simulink model "motor"  (Simulink 8.6)
settings: Solver=FixedStepDiscrete  StartTime=0.0  StopTime=inf  FixedStep=0.002  RelTol=1e-3
PostLoadFcn:
  | ,try, rti_mdl_postloadfcn(bdroot, 'UpdateModel', 160, 'rti1104'); catch, disp(lasterr); end,
undefined symbols (not defined in the file): DiscIntNeverNeededParam
libraries: simulink x3
(part 2 of 3)

== system motor/Chart/Motor_XHHY/Control_HP ==
  In_HP : Inport
  Discrete-Time Integrator : DiscreteIntegrator  InitialConditionSetting=State (most efficient)  SampleTime=-1  ICPrevOutput=DiscIntNeverNeededParam  ICPrevScaledInput=DiscIntNeverNeededParam
  KD_KG : Gain  Gain=0
  P_KP : DataStoreRead  DataStoreName=P_KP
  Product : Product
  Sum : Sum  Inputs=|+-
  Sum1 : Sum  Inputs=|++
  ZP_KN : Gain  Gain=100
  ZP_Kp1 : Gain
  ZP_Kp2 : Gain  Gain=0.001
  ZV_KD1 : Gain  Gain=0.036
  Out_HP : Outport
  wires:
  Product/1 -> ZP_Kp1/1, ZP_Kp2/1
  ZP_Kp2/1 -> ZV_KD1/1
  ZV_KD1/1 -> Sum/1
  Sum/1 -> ZP_KN/1
  Discrete-Time Integrator/1 -> Sum/2
  ZP_Kp1/1 -> Sum1/1
  Sum1/1 -> Out_HP/1
  KD_KG/1 -> Sum1/2
  ZP_KN/1 -> Discrete-Time Integrator/1, KD_KG/1
  In_HP/1 -> Product/1
  P_KP/1 -> Product/2

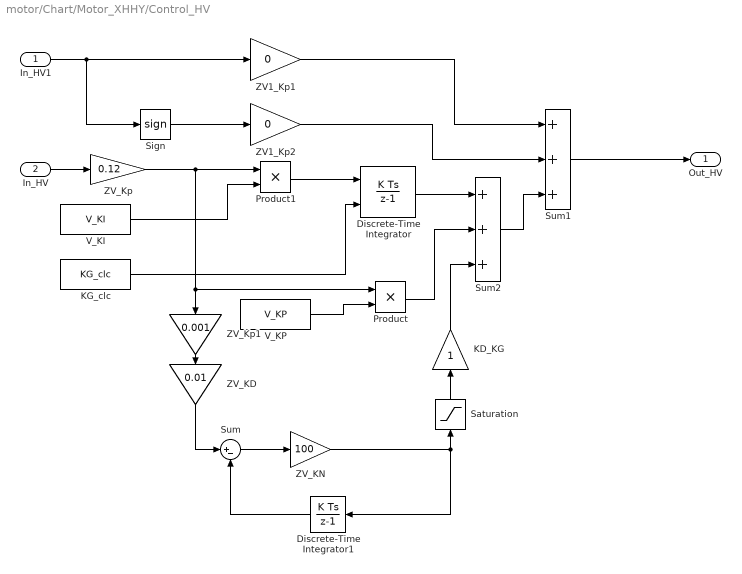
== system motor/Chart/Motor_XHHY/Control_HV ==
  In_HV1 : Inport
  In_HV : Inport  Port=2
  Discrete-Time Integrator : DiscreteIntegrator  ExternalReset=either  SampleTime=-1  SaturateOnIntegerOverflow=on  LimitOutput=on  UpperSaturationLimit=2000  LowerSaturationLimit=-2000  ICPrevOutput=DiscIntNeverNeededParam  ICPrevScaledInput=DiscIntNeverNeededParam
  Discrete-Time Integrator1 : DiscreteIntegrator  InitialConditionSetting=State (most efficient)  SampleTime=-1  LimitOutput=on  UpperSaturationLimit=2000  LowerSaturationLimit=-2000  ICPrevOutput=DiscIntNeverNeededParam  ICPrevScaledInput=DiscIntNeverNeededParam
  KD_KG : Gain
  KG_clc : DataStoreRead  DataStoreName=KG_clc
  Product : Product
  Product1 : Product
  Saturation : Saturate  UpperLimit=300  LowerLimit=-300
  Sign : Signum
  Sum : Sum  Inputs=|+-
  Sum1 : Sum  Inputs=+++
  Sum2 : Sum  Inputs=+++
  V_KI : DataStoreRead  DataStoreName=V_KI
  V_KP : DataStoreRead  DataStoreName=V_KP
  ZV1_Kp1 : Gain  Gain=0
  ZV1_Kp2 : Gain  Gain=0
  ZV_KD : Gain  Gain=0.01
  ZV_KN : Gain  Gain=100
  ZV_Kp : Gain  Gain=0.12
  ZV_Kp1 : Gain  Gain=0.001
  Out_HV : Outport
  wires:
  Product/1 -> Sum2/2
  Discrete-Time Integrator/1 -> Sum2/1
  In_HV/1 -> ZV_Kp/1
  Sign/1 -> ZV1_Kp2/1
  In_HV1/1 -> Sign/1, ZV1_Kp1/1
  Sum1/1 -> Out_HV/1
  Sum2/1 -> Sum1/3
  ZV1_Kp2/1 -> Sum1/2
  ZV1_Kp1/1 -> Sum1/1
  ZV_Kp1/1 -> ZV_KD/1
  ZV_KD/1 -> Sum/1
  Sum/1 -> ZV_KN/1
  Discrete-Time Integrator1/1 -> Sum/2
  ZV_KN/1 -> Discrete-Time Integrator1/1, Saturation/1
  Saturation/1 -> KD_KG/1
  KD_KG/1 -> Sum2/3
  KG_clc/1 -> Discrete-Time Integrator/2
  Product1/1 -> Discrete-Time Integrator/1
  ZV_Kp/1 -> ZV_Kp1/1, Product/1, Product1/1
  V_KP/1 -> Product/2
  V_KI/1 -> Product1/2

== system motor/Chart/Motor_XHHY/If Action Subsystem1 ==
  Action Port : ActionPort  ActionType=elseif
  Data Store Read : DataStoreRead  DataStoreName=JD_XHHY_HC
  Data Store Write1 : DataStoreWrite  DataStoreName=JD_XHHY
  wires:
  Data Store Read/1 -> Data Store Write1/1

== system motor/Chart/Motor_XHHY/If Action Subsystem2 ==
  In1 : Inport
  Action Port : ActionPort  ActionType=else
  Data Store Write : DataStoreWrite  DataStoreName=JD_XHHY_HC
  Data Store Write1 : DataStoreWrite  DataStoreName=JD_XHHY
  wires:
  In1/1 -> Data Store Write/1, Data Store Write1/1

== system motor/Chart/Motor_XHHY/If Action Subsystem3 ==
  In1 : Inport
  Action Port : ActionPort  ActionType=then
  Data Store Write : DataStoreWrite  DataStoreName=JD_XHHY_HC
  Data Store Write1 : DataStoreWrite  DataStoreName=JD_XHHY
  wires:
  In1/1 -> Data Store Write/1, Data Store Write1/1

== system motor/Chart/Motor_XHHY/Switch Case Action Subsystem ==
  In1 : Inport
  Action Port : ActionPort  ActionType=then
  Constant : Constant  Value=0
  Data Store Write : DataStoreWrite  DataStoreName=Angle_extern
  Data Store Write1 : DataStoreWrite  DataStoreName=Angle_internal
  wires:
  In1/1 -> Data Store Write/1
  Constant/1 -> Data Store Write1/1

== system motor/Chart/Motor_XHHY/Switch Case Action Subsystem1 ==
  In1 : Inport
  Action Port : ActionPort  ActionType=else
  Constant : Constant  Value=0
  Data Store Write : DataStoreWrite  DataStoreName=Angle_extern
  Data Store Write1 : DataStoreWrite  DataStoreName=Angle_internal
  wires:
  In1/1 -> Data Store Write1/1
  Constant/1 -> Data Store Write/1

== system motor/Chart/Motor_XHHY/ZYDX_XHHY ==
  Hl : Inport  OutDataTypeStr=double
  Zl : Inport  Port=2  OutDataTypeStr=double
  Fcn1 : Fcn  Expr=u+265.5
  Fcn10 : Fcn  Expr=u*u+1
  Fcn11 : Fcn  Expr=sqrt(u)
  Fcn12 : Fcn  Expr=2*atan(u)
  Fcn2 : Fcn  Expr=(90490.25-u*u)/(20000)
  Fcn3 : Fcn  Expr=(2.655-sqrt(2.655*2.655-u*u+1))/(u+1)
  Fcn4 : Fcn  Expr=2.655*cos(u)
  Fcn5 : Fcn  Expr=u+265.5
  Fcn6 : Fcn  Expr=2*atan(u)
  Fcn7 : Fcn  Expr=(90490.25-u*u)/(20000)
  Fcn8 : Fcn  Expr=u*u
  Fcn9 : Fcn  Expr=1/(u+1)
  Product : Product  RndMeth=Zero
  Sum2 : Sum  Inputs=|+-
  Sum3 : Sum  Inputs=|+-
  Hq : Outport
  wires:
  Fcn11/1 -> Sum2/2
  Fcn4/1 -> Fcn10/1, Sum2/1
  Fcn3/1 -> Fcn6/1
  Hl/1 -> Fcn5/1
  Fcn1/1 -> Fcn2/1
  Product/1 -> Fcn12/1
  Fcn12/1 -> Hq/1
  Fcn2/1 -> Fcn3/1
  Fcn7/1 -> Fcn9/1, Fcn8/1
  Fcn6/1 -> Fcn4/1
  Zl/1 -> Fcn1/1
  Sum2/1 -> Product/1
  Fcn10/1 -> Sum3/1
  Fcn5/1 -> Fcn7/1
  Sum3/1 -> Fcn11/1
  Fcn9/1 -> Product/2
  Fcn8/1 -> Sum3/2

== system motor/Chart/Motor_XHZY/Control_ZP ==
  In_ZP : Inport
  Discrete-Time Integrator : DiscreteIntegrator  InitialConditionSetting=State (most efficient)  SampleTime=-1  ICPrevOutput=DiscIntNeverNeededParam  ICPrevScaledInput=DiscIntNeverNeededParam
  KD_KG : Gain  Gain=0
  P_KP : DataStoreRead  DataStoreName=P_KP
  Product : Product
  Sum : Sum  Inputs=|+-
  Sum1 : Sum  Inputs=|++
  ZP_KN : Gain  Gain=100
  ZP_Kp1 : Gain
  ZP_Kp2 : Gain  Gain=0.001
  ZV_KD1 : Gain  Gain=0.036
  Out_ZP : Outport
  wires:
  Product/1 -> ZP_Kp1/1, ZP_Kp2/1
  ZP_Kp2/1 -> ZV_KD1/1
  ZV_KD1/1 -> Sum/1
  Sum/1 -> ZP_KN/1
  Discrete-Time Integrator/1 -> Sum/2
  ZP_Kp1/1 -> Sum1/1
  Sum1/1 -> Out_ZP/1
  KD_KG/1 -> Sum1/2
  ZP_KN/1 -> Discrete-Time Integrator/1, KD_KG/1
  In_ZP/1 -> Product/1
  P_KP/1 -> Product/2

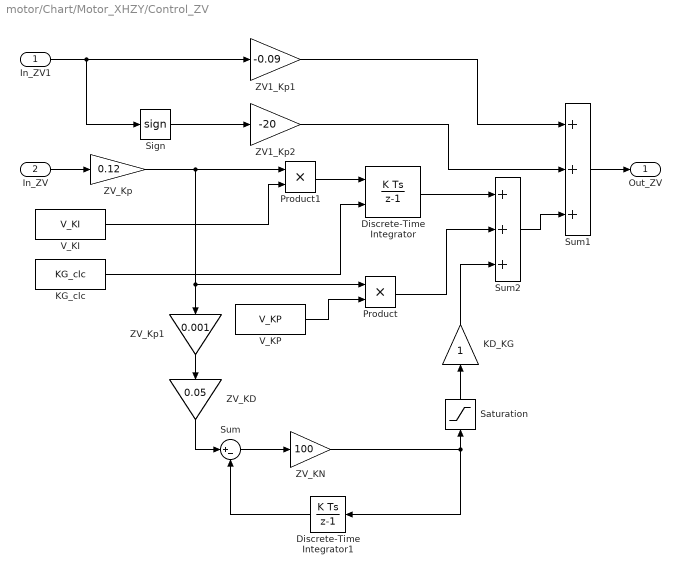
== system motor/Chart/Motor_XHZY/Control_ZV ==
  In_ZV1 : Inport
  In_ZV : Inport  Port=2
  Discrete-Time Integrator : DiscreteIntegrator  ExternalReset=either  SampleTime=-1  SaturateOnIntegerOverflow=on  LimitOutput=on  UpperSaturationLimit=2000  LowerSaturationLimit=-2000  ICPrevOutput=DiscIntNeverNeededParam  ICPrevScaledInput=DiscIntNeverNeededParam
  Discrete-Time Integrator1 : DiscreteIntegrator  InitialConditionSetting=State (most efficient)  SampleTime=-1  ICPrevOutput=DiscIntNeverNeededParam  ICPrevScaledInput=DiscIntNeverNeededParam
  KD_KG : Gain
  KG_clc : DataStoreRead  DataStoreName=KG_clc
  Product : Product
  Product1 : Product
  Saturation : Saturate  UpperLimit=300  LowerLimit=-300
  Sign : Signum
  Sum : Sum  Inputs=|+-
  Sum1 : Sum  Inputs=+++
  Sum2 : Sum  Inputs=+++
  V_KI : DataStoreRead  DataStoreName=V_KI
  V_KP : DataStoreRead  DataStoreName=V_KP
  ZV1_Kp1 : Gain  Gain=-0.09
  ZV1_Kp2 : Gain  Gain=-20
  ZV_KD : Gain  Gain=0.05
  ZV_KN : Gain  Gain=100
  ZV_Kp : Gain  Gain=0.12
  ZV_Kp1 : Gain  Gain=0.001
  Out_ZV : Outport
  wires:
  Product/1 -> Sum2/2
  Discrete-Time Integrator/1 -> Sum2/1
  In_ZV/1 -> ZV_Kp/1
  Sign/1 -> ZV1_Kp2/1
  In_ZV1/1 -> Sign/1, ZV1_Kp1/1
  Sum1/1 -> Out_ZV/1
  Sum2/1 -> Sum1/3
  ZV1_Kp2/1 -> Sum1/2
  ZV1_Kp1/1 -> Sum1/1
  ZV_Kp1/1 -> ZV_KD/1
  ZV_KD/1 -> Sum/1
  Sum/1 -> ZV_KN/1
  Discrete-Time Integrator1/1 -> Sum/2
  ZV_KN/1 -> Discrete-Time Integrator1/1, Saturation/1
  Saturation/1 -> KD_KG/1
  KD_KG/1 -> Sum2/3
  KG_clc/1 -> Discrete-Time Integrator/2
  Product1/1 -> Discrete-Time Integrator/1
  ZV_Kp/1 -> ZV_Kp1/1, Product/1, Product1/1
  V_KP/1 -> Product/2
  V_KI/1 -> Product1/2

== system motor/Chart/Motor_XHZY/If Action Subsystem1 ==
  Action Port : ActionPort  ActionType=elseif
  Data Store Read : DataStoreRead  DataStoreName=JD_XHZY_HC
  Data Store Read1 : DataStoreRead  DataStoreName=YJ_XHZY_HC
  Data Store Write1 : DataStoreWrite  DataStoreName=JD_XHZY
  Data Store Write2 : DataStoreWrite  DataStoreName=YJ_XHZY
  wires:
  Data Store Read/1 -> Data Store Write1/1
  Data Store Read1/1 -> Data Store Write2/1

== system motor/Chart/Motor_XHZY/If Action Subsystem2 ==
  In1 : Inport
  In2 : Inport  Port=2
  Action Port : ActionPort  ActionType=else
  Data Store Write : DataStoreWrite  DataStoreName=JD_XHZY_HC
  Data Store Write1 : DataStoreWrite  DataStoreName=JD_XHZY
  Data Store Write2 : DataStoreWrite  DataStoreName=YJ_XHZY_HC
  Data Store Write3 : DataStoreWrite  DataStoreName=YJ_XHZY
  wires:
  In1/1 -> Data Store Write/1, Data Store Write1/1
  In2/1 -> Data Store Write3/1, Data Store Write2/1

== system motor/Chart/Motor_XHZY/If Action Subsystem3 ==
  In1 : Inport
  In2 : Inport  Port=2
  Action Port : ActionPort  ActionType=then
  Data Store Write : DataStoreWrite  DataStoreName=JD_XHZY_HC
  Data Store Write1 : DataStoreWrite  DataStoreName=JD_XHZY
  Data Store Write2 : DataStoreWrite  DataStoreName=YJ_XHZY_HC
  Data Store Write3 : DataStoreWrite  DataStoreName=YJ_XHZY
  wires:
  In1/1 -> Data Store Write/1, Data Store Write1/1
  In2/1 -> Data Store Write3/1, Data Store Write2/1

== system motor/Chart/Motor_XHZY/Switch Case Action Subsystem ==
  In1 : Inport
  Action Port : ActionPort  ActionType=then
  Constant : Constant  Value=0
  Data Store Write : DataStoreWrite  DataStoreName=Angle_extern
  Data Store Write1 : DataStoreWrite  DataStoreName=Angle_internal
  wires:
  In1/1 -> Data Store Write/1
  Constant/1 -> Data Store Write1/1

== system motor/Chart/Motor_XHZY/Switch Case Action Subsystem1 ==
  In1 : Inport
  Action Port : ActionPort  ActionType=else
  Constant : Constant  Value=0
  Data Store Write : DataStoreWrite  DataStoreName=Angle_extern
  Data Store Write1 : DataStoreWrite  DataStoreName=Angle_internal
  wires:
  In1/1 -> Data Store Write1/1
  Constant/1 -> Data Store Write/1

== system motor/Chart/Motor_XHZY/ZYDX_XHZY ==
  Zl : Inport
  Fcn1 : Fcn  Expr=u+265.5
  Fcn2 : Fcn  Expr=(90490.25-u*u)/(20000)
  Fcn3 : Fcn  Expr=(2.655-sqrt(2.655*2.655-u*u+1))/(u+1)
  Fcn6 : Fcn  Expr=2*atan(u)
  Zq : Outport
  wires:
  Fcn3/1 -> Fcn6/1
  Zl/1 -> Fcn1/1
  Fcn6/1 -> Zq/1
  Fcn1/1 -> Fcn2/1
  Fcn2/1 -> Fcn3/1

== system motor/Chart/Open_Motor/sudu_PI ==
  In_ZV : Inport
  Discrete-Time Integrator : DiscreteIntegrator  ExternalReset=either  SampleTime=-1  SaturateOnIntegerOverflow=on  LimitOutput=on  UpperSaturationLimit=1000  LowerSaturationLimit=-1000  ICPrevOutput=DiscIntNeverNeededParam  ICPrevScaledInput=DiscIntNeverNeededParam
  Discrete-Time Integrator1 : DiscreteIntegrator  InitialConditionSetting=State (most efficient)  SampleTime=-1  ICPrevOutput=DiscIntNeverNeededParam  ICPrevScaledInput=DiscIntNeverNeededParam
  KD_KG : Gain  Gain=0
  KG_clc : DataStoreRead  DataStoreName=KG_clc
  Saturation : Saturate  UpperLimit=300  LowerLimit=-300
  Sum : Sum  Inputs=|+-
  Sum2 : Sum  Inputs=|+++
  ZV_KD : Gain  Gain=0.095
  ZV_KN : Gain  Gain=100
  ZV_Ki : Gain  Gain=0
  ZV_Kp : Gain  Gain=0.7
  ZV_Kp1 : Gain  Gain=0.001
  ZV_Kpt : Gain
  Out_ZV : Outport
  wires:
  ZV_Kpt/1 -> Sum2/2
  Discrete-Time Integrator/1 -> Sum2/1
  In_ZV/1 -> ZV_Kp/1
  ZV_Kp/1 -> ZV_Ki/1, ZV_Kp1/1, ZV_Kpt/1
  Sum2/1 -> Out_ZV/1
  ZV_Kp1/1 -> ZV_KD/1
  ZV_KD/1 -> Sum/1
  Sum/1 -> ZV_KN/1
  Discrete-Time Integrator1/1 -> Sum/2
  ZV_KN/1 -> Saturation/1, Discrete-Time Integrator1/1
  Saturation/1 -> KD_KG/1
  KD_KG/1 -> Sum2/3
  KG_clc/1 -> Discrete-Time Integrator/2
  ZV_Ki/1 -> Discrete-Time Integrator/1

== system motor/Chart/Waveform_Build/If Action Subsystem1 ==
  In1 : Inport
  In2 : Inport  Port=2
  Action Port : ActionPort  ActionType=then
  Data Store Read5 : DataStoreRead  DataStoreName=T_Count
  Data Store Write1 : DataStoreWrite  DataStoreName=T_Count
  Data Store Write2 : DataStoreWrite  DataStoreName=Temp1
  Data Store Write3 : DataStoreWrite  DataStoreName=T
  MATLAB Function : MATLAB Function  TreatAsAtomicUnit=on
  Out1 : Outport
  wires:
  In1/1 -> Out1/1
  In2/1 -> Data Store Write2/1
  MATLAB Function/1(y1) -> Data Store Write3/1
  Data Store Read5/1 -> MATLAB Function/1(u)
  MATLAB Function/2(y2) -> Data Store Write1/1

== system motor/Chart/Waveform_Build/If Action Subsystem2 ==
  In1 : Inport
  In2 : Inport  Port=2
  Action Port : ActionPort  ActionType=then
  Data Store Write2 : DataStoreWrite  DataStoreName=Temp2
  Out1 : Outport
  wires:
  In2/1 -> Data Store Write2/1
  In1/1 -> Out1/1

== system motor/Chart/Waveform_Build/If Action Subsystem3 ==
  Action Port : ActionPort  ActionType=else
  Add20 : Sum
  Constant3 : Constant
  Data Store Read5 : DataStoreRead  DataStoreName=T_Count
  Data Store Write1 : DataStoreWrite  DataStoreName=T_Count
  Saturation : Saturate  UpperLimit=999  LowerLimit=0
  Scope4 : Scope
  wires:
  Add20/1 -> Saturation/1
  Data Store Read5/1 -> Add20/1
  Constant3/1 -> Add20/2
  Saturation/1 -> Scope4/1, Data Store Write1/1

== system motor/Chart/Waveform_Build/If Action Subsystem4 ==
  In1 : Inport
  Action Port : ActionPort  ActionType=then
  Out1 : Outport
  wires:
  In1/1 -> Out1/1

== system motor/Chart/Angle_Calculation/If Action Subsystem1/ZYDX_HYDG ==
  l2 : Inport
  Cl1 : Fcn  Expr=(2*0.1*0.1+0.2655*0.2655-u*u)/(2*0.1*0.1)
  Fcn : Fcn  Expr=(2.655-sqrt(2.655*2.655-u*u+1))/(u+1)
  Fcn4 : Fcn  Expr=2*atan(u)
  Fcn7 : Fcn  Expr=u+0.2655
  x : Outport
  wires:
  Fcn4/1 -> x/1
  l2/1 -> Fcn7/1
  Fcn/1 -> Fcn4/1
  Fcn7/1 -> Cl1/1
  Cl1/1 -> Fcn/1

== system motor/Chart/Angle_Calculation/If Action Subsystem2/ZYDX_XHZY ==
  Zl : Inport
  Fcn1 : Fcn  Expr=u+265.5
  Fcn2 : Fcn  Expr=(90490.25-u*u)/(20000)
  Fcn3 : Fcn  Expr=(2.655-sqrt(2.655*2.655-u*u+1))/(u+1)
  Fcn6 : Fcn  Expr=2*atan(u)
  Zq : Outport
  wires:
  Fcn3/1 -> Fcn6/1
  Zl/1 -> Fcn1/1
  Fcn6/1 -> Zq/1
  Fcn1/1 -> Fcn2/1
  Fcn2/1 -> Fcn3/1

== system motor/Chart/Angle_Calculation/If Action Subsystem3/ZYDX_XHHY ==
  Hl : Inport  OutDataTypeStr=double
  Zl : Inport  Port=2  OutDataTypeStr=double
  Fcn1 : Fcn  Expr=u+265.5
  Fcn10 : Fcn  Expr=u*u+1
  Fcn11 : Fcn  Expr=sqrt(u)
  Fcn12 : Fcn  Expr=2*atan(u)
  Fcn2 : Fcn  Expr=(90490.25-u*u)/(20000)
  Fcn3 : Fcn  Expr=(2.655-sqrt(2.655*2.655-u*u+1))/(u+1)
  Fcn4 : Fcn  Expr=2.655*cos(u)
  Fcn5 : Fcn  Expr=u+265.5
  Fcn6 : Fcn  Expr=2*atan(u)
  Fcn7 : Fcn  Expr=(90490.25-u*u)/(20000)
  Fcn8 : Fcn  Expr=u*u
  Fcn9 : Fcn  Expr=1/(u+1)
  Product : Product  RndMeth=Zero
  Sum2 : Sum  Inputs=|+-
  Sum3 : Sum  Inputs=|+-
  Hq : Outport
  wires:
  Fcn11/1 -> Sum2/2
  Fcn4/1 -> Fcn10/1, Sum2/1
  Fcn3/1 -> Fcn6/1
  Hl/1 -> Fcn5/1
  Fcn1/1 -> Fcn2/1
  Product/1 -> Fcn12/1
  Fcn12/1 -> Hq/1
  Fcn2/1 -> Fcn3/1
  Fcn7/1 -> Fcn9/1, Fcn8/1
  Fcn6/1 -> Fcn4/1
  Zl/1 -> Fcn1/1
  Sum2/1 -> Product/1
  Fcn10/1 -> Sum3/1
  Fcn5/1 -> Fcn7/1
  Sum3/1 -> Fcn11/1
  Fcn9/1 -> Product/2
  Fcn8/1 -> Sum3/2

== system motor/Chart/Angle_Calculation_HY/fs_plat/ZYDX_HYDG ==
  l2 : Inport
  Cl1 : Fcn  Expr=(2*0.1*0.1+0.2655*0.2655-u*u)/(2*0.1*0.1)
  Fcn : Fcn  Expr=(2.655-sqrt(2.655*2.655-u*u+1))/(u+1)
  Fcn4 : Fcn  Expr=2*atan(u)
  Fcn7 : Fcn  Expr=u+0.2655
  x : Outport
  wires:
  Fcn4/1 -> x/1
  l2/1 -> Fcn7/1
  Fcn/1 -> Fcn4/1
  Fcn7/1 -> Cl1/1
  Cl1/1 -> Fcn/1

== system motor/Chart/BJ/If Action Subsystem/If Action Subsystem ==
  Action Port : ActionPort  ActionType=then
  Data Store Write : DataStoreWrite  DataStoreName=PC1
  Data Store Write1 : DataStoreWrite  DataStoreName=PC2
  Data Type Conversion : DataTypeConversion  OutDataTypeStr=boolean
  Pulse Generator : DiscretePulseGenerator  Period=500  PulseWidth=250  SampleTime=-1
  wires:
  Pulse Generator/1 -> Data Type Conversion/1
  Data Type Conversion/1 -> Data Store Write1/1, Data Store Write/1

== system motor/Chart/BJ/If Action Subsystem/If Action Subsystem1 ==
  Action Port : ActionPort  ActionType=elseif
  Constant : Constant  OutDataTypeStr=boolean
  Data Store Write : DataStoreWrite  DataStoreName=PC1
  Data Store Write1 : DataStoreWrite  DataStoreName=PC2
  Data Type Conversion : DataTypeConversion  OutDataTypeStr=boolean
  Pulse Generator : DiscretePulseGenerator  Period=500  PulseWidth=250  SampleTime=-1
  wires:
  Pulse Generator/1 -> Data Type Conversion/1
  Data Type Conversion/1 -> Data Store Write/1
  Constant/1 -> Data Store Write1/1

== system motor/Chart/BJ/If Action Subsystem/If Action Subsystem2 ==
  Action Port : ActionPort  ActionType=else
  Constant : Constant  OutDataTypeStr=boolean
  Constant1 : Constant  Value=0  OutDataTypeStr=boolean
  Data Store Write : DataStoreWrite  DataStoreName=PC1
  Data Store Write1 : DataStoreWrite  DataStoreName=PC2
  wires:
  Constant/1 -> Data Store Write/1
  Constant1/1 -> Data Store Write1/1

== system motor/Chart/BJ/If Action Subsystem1/If Action Subsystem ==
  Action Port : ActionPort  ActionType=then
  Data Store Write : DataStoreWrite  DataStoreName=PC1
  Data Store Write1 : DataStoreWrite  DataStoreName=PC2
  Data Type Conversion : DataTypeConversion  OutDataTypeStr=boolean
  Pulse Generator : DiscretePulseGenerator  Period=500  PulseWidth=250  SampleTime=-1
  wires:
  Pulse Generator/1 -> Data Type Conversion/1
  Data Type Conversion/1 -> Data Store Write1/1, Data Store Write/1

== system motor/Chart/BJ/If Action Subsystem1/If Action Subsystem1 ==
  Action Port : ActionPort  ActionType=elseif
  Constant : Constant  OutDataTypeStr=boolean
  Data Store Write : DataStoreWrite  DataStoreName=PC1
  Data Store Write1 : DataStoreWrite  DataStoreName=PC2
  Data Type Conversion : DataTypeConversion  OutDataTypeStr=boolean
  Pulse Generator : DiscretePulseGenerator  Period=500  PulseWidth=250  SampleTime=-1
  wires:
  Pulse Generator/1 -> Data Type Conversion/1
  Data Type Conversion/1 -> Data Store Write/1
  Constant/1 -> Data Store Write1/1

== system motor/Chart/BJ/If Action Subsystem1/If Action Subsystem2 ==
  Action Port : ActionPort  ActionType=else
  Constant : Constant  OutDataTypeStr=boolean
  Data Store Write : DataStoreWrite  DataStoreName=PC2
  Data Store Write1 : DataStoreWrite  DataStoreName=PC1
  Data Type Conversion : DataTypeConversion  OutDataTypeStr=boolean
  Pulse Generator : DiscretePulseGenerator  Period=500  PulseWidth=250  SampleTime=-1
  wires:
  Pulse Generator/1 -> Data Type Conversion/1
  Data Type Conversion/1 -> Data Store Write/1
  Constant/1 -> Data Store Write1/1

== system motor/Chart/BJ/If Action Subsystem2/If Action Subsystem ==
  Action Port : ActionPort  ActionType=then
  Data Store Write : DataStoreWrite  DataStoreName=PC1
  Data Store Write1 : DataStoreWrite  DataStoreName=PC2
  Data Type Conversion : DataTypeConversion  OutDataTypeStr=boolean
  Pulse Generator : DiscretePulseGenerator  Period=500  PulseWidth=250  SampleTime=-1
  wires:
  Pulse Generator/1 -> Data Type Conversion/1
  Data Type Conversion/1 -> Data Store Write1/1, Data Store Write/1

== system motor/Chart/BJ/If Action Subsystem2/If Action Subsystem1 ==
  Action Port : ActionPort  ActionType=elseif
  Constant : Constant  OutDataTypeStr=boolean
  Data Store Write : DataStoreWrite  DataStoreName=PC1
  Data Store Write1 : DataStoreWrite  DataStoreName=PC2
  Data Type Conversion : DataTypeConversion  OutDataTypeStr=boolean
  Pulse Generator : DiscretePulseGenerator  Period=500  PulseWidth=250  SampleTime=-1
  wires:
  Pulse Generator/1 -> Data Type Conversion/1
  Data Type Conversion/1 -> Data Store Write/1
  Constant/1 -> Data Store Write1/1

== system motor/Chart/BJ/If Action Subsystem2/If Action Subsystem2 ==
  Action Port : ActionPort  ActionType=else
  Constant : Constant  OutDataTypeStr=boolean
  Constant1 : Constant  Value=0  OutDataTypeStr=boolean
  Data Store Write : DataStoreWrite  DataStoreName=PC1
  Data Store Write1 : DataStoreWrite  DataStoreName=PC2
  wires:
  Constant/1 -> Data Store Write/1
  Constant1/1 -> Data Store Write1/1

== system motor/Chart/Motor_HYDG/fs_plat/ZYDX_HYDG ==
  l2 : Inport
  Cl1 : Fcn  Expr=(2*0.1*0.1+0.2655*0.2655-u*u)/(2*0.1*0.1)
  Fcn : Fcn  Expr=(2.655-sqrt(2.655*2.655-u*u+1))/(u+1)
  Fcn4 : Fcn  Expr=2*atan(u)
  Fcn7 : Fcn  Expr=u+0.2655
  x : Outport
  wires:
  Fcn4/1 -> x/1
  l2/1 -> Fcn7/1
  Fcn/1 -> Fcn4/1
  Fcn7/1 -> Cl1/1
  Cl1/1 -> Fcn/1

== matlab function Chart/Waveform_Build/If Action Subsystem1/MATLAB Function ==
  data: u input double; y1 output double; y2 output double
function [y1,y2] = fcn(u)
%#codegen

y1 = u + 1;
y2 = 0;
